simulink model "System_Design_Quadrocopter"  (Simulink 7.5)
settings: Solver=ode45  StartTime=0.0  StopTime=30  RelTol=1e-3
model workspace (MAT data in the model file):
  System_Design_Quadrocopter_optim : srogui.SimProjectForm (value not decoded)
values from neighbouring files (symbols this model uses):
  phi0 = 0.15    [Quadrocopter_control_Driver.m]    (also in calc_stability.m = 0)
  r_phi0 = 0    [Quadrocopter_control_Driver.m]    (also in calc_stability.m)
  r_psi0 = 0    [Quadrocopter_control_Driver.m]    (also in calc_stability.m)
  r_theta0 = 0    [Quadrocopter_control_Driver.m]    (also in calc_stability.m)
  theta0 = 0.15    [Quadrocopter_control_Driver.m]    (also in calc_stability.m = 0)
  Ts = 0.01    [Reglerauslegung.m]    (also in Test_Reglerauslegung.m)
undefined symbols (not defined in the file or in its folder): bodyCtrl_phiCtrl_KD, bodyCtrl_phiCtrl_KI, bodyCtrl_phiCtrl_KP, bodyCtrl_rphiCtrl_KD, bodyCtrl_rphiCtrl_KI, bodyCtrl_rphiCtrl_KP, bodyCtrl_rpsiCtrl_KD, bodyCtrl_rpsiCtrl_KI, bodyCtrl_rpsiCtrl_KP, bodyCtrl_rthetaCtrl_KD, bodyCtrl_rthetaCtrl_KI, bodyCtrl_rthetaCtrl_KP, bodyCtrl_thetaCtrl_KD, bodyCtrl_thetaCtrl_KI, bodyCtrl_thetaCtrl_KP, boom, f1, f2, f3, f4, f5, g, I_x, I_y, I_z, m, positionCtrl_rpsiCtrl_KD, positionCtrl_rpsiCtrl_KI, positionCtrl_rpsiCtrl_KP, sigbuilder_block, speed, thrust, Ts_Opt
libraries: simulink x39, dspobslib x4, Copter_Library x3, Control_lib x1, sdolib x1
(part 1 of 4)
CloseFcn:
  | rtwprivate ssgensfun ModelCloseRequest System_Design_Quadrocopter
settings Model: Creator=roczit00  LastModifiedBy=Anonymos  BufferReuse=off
settings DataIOCC: LimitDataPoints=off
settings OptimizationCC: BlockReduction=off  InlineParams=on  BufferReuse=off
settings DebuggingCC: AlgebraicLoopMsg=none  SolverPrmCheckMsg=none  UnconnectedInputMsg=none  UnconnectedOutputMsg=none  UnconnectedLineMsg=none  StrictBusMsg=Warning

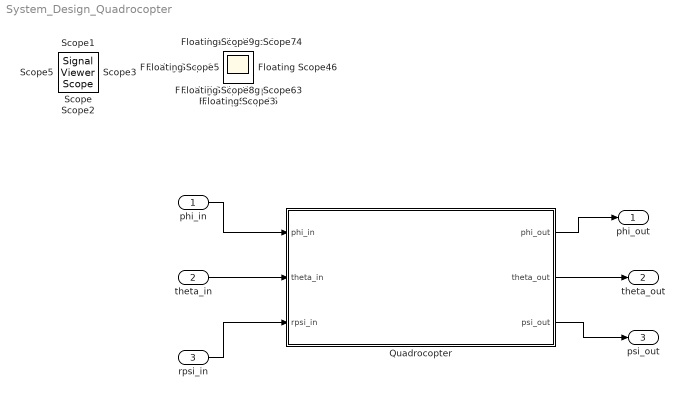
== system System_Design_Quadrocopter ==
  phi_in : Inport  OutDataType=fixdt(1, 16)  OutScaling=2^0
  theta_in : Inport  Port=2  OutDataType=fixdt(1, 16)  OutScaling=2^0
  rpsi_in : Inport  Port=3  OutDataType=fixdt(1, 16)  OutScaling=2^0
  Quadrocopter : Subsystem
  phi_out : Outport  OutDataType=fixdt(1, 16)  OutScaling=2^0
  theta_out : Outport  Port=2  OutDataType=fixdt(1, 16)  OutScaling=2^0
  psi_out : Outport  Port=3  OutDataType=fixdt(1, 16)  OutScaling=2^0
  Floating Scope{,1..18} (19 alike) : Scope
      Floating Scope settings: Floating=on  YMin=-40  YMax=90
      Floating Scope1 settings: Floating=on
      Floating Scope10 settings: Floating=on  SaveName=ScopeData12
      Floating Scope11 settings: Floating=on  SaveName=ScopeData13
      Floating Scope12 settings: Floating=on  YMin=-2500  YMax=27500  SaveName=ScopeData14
      Floating Scope13 settings: Floating=on  YMin=0  YMax=0.3  SaveName=ScopeData15
      Floating Scope14 settings: Floating=on  SaveName=ScopeData8
      Floating Scope15 settings: Floating=on  SaveName=ScopeData9
      Floating Scope16 settings: Floating=on  YMin=-0.35  YMax=0.15  SaveName=ScopeData16
      Floating Scope17 settings: Floating=on  YMin=0.1  YMax=0.55  SaveName=ScopeData17
      Floating Scope18 settings: Floating=on  SaveName=ScopeData18
      Floating Scope2 settings: Floating=on  YMin=-6000  YMax=2500  SaveName=ScopeData2
      Floating Scope3 settings: Floating=on  SaveName=ScopeData3
      Floating Scope4 settings: Floating=on  SaveName=ScopeData4
      Floating Scope5 settings: Floating=on  YMin=-0.7  YMax=0.8  SaveName=ScopeData5
      Floating Scope6 settings: Floating=on  YMin=-1  YMax=1  SaveName=ScopeData6
      Floating Scope7 settings: Floating=on  YMin=-15  YMax=10  SaveName=ScopeData7
      Floating Scope8 settings: Floating=on  YMax=45  SaveName=ScopeData10
      Floating Scope9 settings: Floating=on  YMin=-7  YMax=9  SaveName=ScopeData11
  Scope{,1..3,5} (5 alike) : SignalViewerScope  IOType=viewer  RefreshTime=0.035000
      Scope settings: YMin=-0.01  YMax=0.1
      Scope2 settings: SaveName=ScopeData2
      Scope3 settings: SaveName=ScopeData3
      Scope5 settings: YMin=0  YMax=275  SaveName=ScopeData4
  wires:
  rpsi_in/1 -> Quadrocopter/3(rpsi_in)
  theta_in/1 -> Quadrocopter/2(theta_in)
  phi_in/1 -> Quadrocopter/1(phi_in)
  Quadrocopter/1(phi_out) -> phi_out/1
  Quadrocopter/3(psi_out) -> psi_out/1
  Quadrocopter/2(theta_out) -> theta_out/1

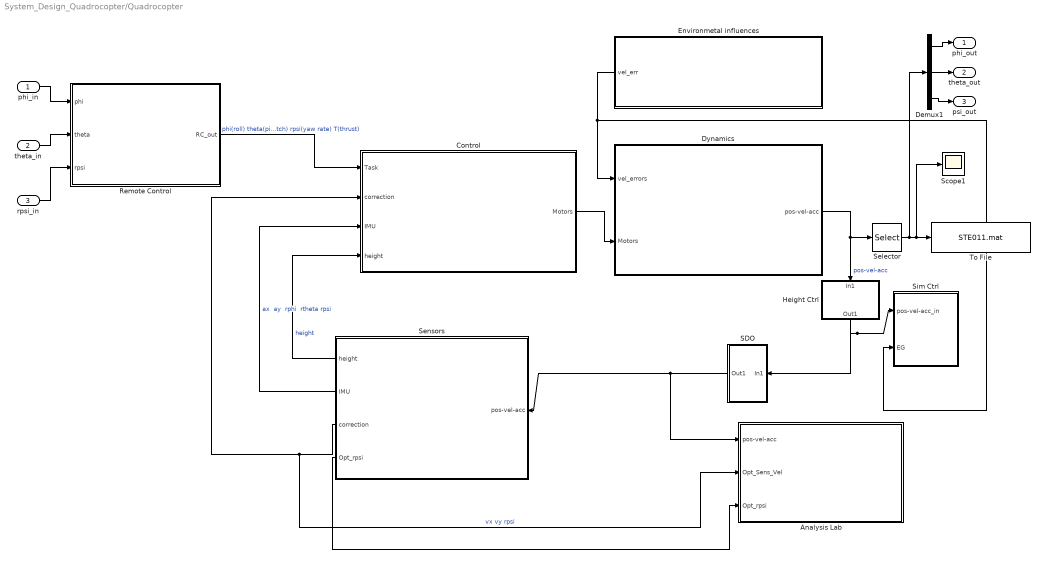
== system System_Design_Quadrocopter/Quadrocopter ==
  phi_in : Inport  OutDataType=fixdt(1, 16)  OutScaling=2^0
  theta_in : Inport  Port=2  OutDataType=fixdt(1, 16)  OutScaling=2^0
  rpsi_in : Inport  Port=3  OutDataType=fixdt(1, 16)  OutScaling=2^0
  Analysis Lab : Subsystem
      mask Display: image(imresize(imread('DecoImg/Lab.jpg'),0.12), 'center');
  Control : Subsystem
      mask Display: image(imresize(imread('DecoImg/Control.jpg'),0.2), 'center');
  Demux1 : Demux  Outputs=3
  Dynamics : Subsystem
      mask Display: image(imresize(imread('DecoImg/Dynamics.jpg'),0.2), 'center');
  Environmetal influences : Subsystem
      mask Display: image(imresize(imread('DecoImg/Environment.jpg'),0.2), 'center');
  Height Ctrl : Subsystem  mask{Step_T=0, Gain=5, Delay=3}
      mask prompts: Step_T "Step Time"; Delay "LP Delay"
  Remote Control : Subsystem
      mask Display: image(imresize(imread('DecoImg/RemoteControl.jpg'),0.3), 'center');
  SDO : Subsystem
  Scope1 : Scope
      settings: YMin=-2  YMax=2  SaveName=ScopeData22
  Selector : Selector  InputPortWidth=pos_vel_acc_dim  IndexOptions=Index vector (dialog)  Indices=[4 5 12]  OutputSizes=1
  Sensors : Subsystem
      mask Display: image(imresize(imread('DecoImg/Sensors.jpg'),0.1), 'center');
  Sim Ctrl : Subsystem  mask{Per_Cent_Gain=0.1, ErrorGain=6}
      mask prompts: Per_Cent_Gain "Per Cent of Gain for threshold"; ErrorGain "Error Gain"
  To File : ToFile  Filename=STE011.mat  MatrixName=Tfile
  phi_out : Outport  OutDataType=fixdt(1, 16)  OutScaling=2^0
  theta_out : Outport  Port=2  OutDataType=fixdt(1, 16)  OutScaling=2^0
  psi_out : Outport  Port=3  OutDataType=fixdt(1, 16)  OutScaling=2^0
  wires:
  Control/1(Motors) -> Dynamics/2(Motors)
  Dynamics/1(pos-vel-acc) -> Height Ctrl/1(In1), Selector/1  "pos-vel-acc"
  Sensors/2(IMU) -> Control/3(IMU)  "ax  ay  rphi  rtheta rpsi"
  Sensors/1(height) -> Control/4(height)  "height"
  Sensors/3(correction) -> Control/2(correction), Analysis Lab/2(Opt_Sens_Vel)  "vx vy rpsi"
  Environmetal influences/1(vel_err) -> Dynamics/1(vel_errors), Sim Ctrl/2(EG)
  Height Ctrl/1(Out1) -> Sim Ctrl/1(pos-vel-acc_in), SDO/1(In1)
  Sensors/4(Opt_rpsi) -> Analysis Lab/3(Opt_rpsi)
  Remote Control/1(RC_out) -> Control/1(Task)  "phi(roll) theta(pitch) rpsi(yaw rate) T(thrust)"
  Selector/1 -> Scope1/1, To File/1, Demux1/1
  SDO/1(Out1) -> Analysis Lab/1(pos-vel-acc), Sensors/1(pos-vel-acc)
  rpsi_in/1 -> Remote Control/3(rpsi)
  theta_in/1 -> Remote Control/2(theta)
  phi_in/1 -> Remote Control/1(phi)
  Demux1/3 -> psi_out/1
  Demux1/2 -> theta_out/1
  Demux1/1 -> phi_out/1

== system System_Design_Quadrocopter/Quadrocopter/Analysis Lab ==
  note: [Time Opt_Vx Opt_Vy Opt_Rpsi Opt_x Opt_y Opt_psi x y z vx vy rpsi]
  pos-vel-acc : Inport
  Opt_Sens_Vel : Inport  Port=2
  Opt_rpsi : Inport  Port=3
  Copter Animation : Subsystem  mask(Quadrocopter Animation){AXES=[-100 100 -100 100 0 100], T_INT=1/25, K_VAR=Feste Position, K_POS=[30 0 6], K_ANGLE=27, A_ON=on, u_phi=on, u_theta=on, u_psi=on, u_x=on, u_y=on, u_z=on}
      mask prompts: AXES "Achsen Grenzen [xmin xmax ymin ymax zmin zmax]"; T_INT "Zeitintervall zwischen Aktualisierungen [s]:"; K_VAR "Kamera Art:"; K_POS "Ort der Kamera [xc yc zc]:"; K_ANGLE "Öffnungswinkel der Kamera [Grad]:"; A_ON "Animation Einschalten:"; u_phi "Use Input phi:"; u_theta "Use Input theta:"; u_psi "Use Input psi:"; u_x "Use Input x:"; u_y "Use Input y:"; u_z "Use Input z:"
      mask help: Erstellt eine 3-D animierte Ansicht eines Quadrocopters.
      mask init:
      | Config.axes = AXES;
      | Config.update = T_INT;
      | Config.camera_view = K_VAR;
      | Config.camera_pos = K_POS;
      | Config.view = K_ANGLE;
      | Config.Animenable = A_ON;
      | Config.phi = u_phi;
      | Config.theta = u_theta;
      | Config.psi = u_psi;
      | Config.x = u_x;
      | Config.y = u_y;
      | Config.z = u_z;
      mask Help:
      | <p>Dieser Block erstellt ein 3 dimensionales Fenster eines Quadrocopters.
      | 
      | <p><H4>Block Eingänge</H4>
      | Der Eingangsvektor bestehend aus:
      | <ul>
      | <li>X-Koordinate - Ort bezogen auf die X-Achse
      | <li>Y-Koordinate - Ort bezogen auf die Y-Achse
      | <li>Z-Koordinate - Ort bezogen auf die Z-Achse
      | <li>Psi - Yaw Drehung um die Z-Achse
      | <li>Phi - Roll Drehen um die Achse in Flugrichtung
      | <li>theta - pitch Neigung in Flugrichtung nach oben bzw. unten
      | </ul></p>
      mask StyleString: edit,edit,popup(Feste Position|Frei bewegbar),edit,edit,checkbox,checkbox,checkbox,checkbox,checkbox,checkbox,checkbox
  Demux : Demux  Outputs=6
  Demux2 : Demux  Outputs=3
  Integrator1 : Integrator
  Integrator2 : Integrator
  Integrator3 : Integrator
  Mux : Mux  Inputs=3
  Mux1 : Mux  Inputs=6
  Mux3 : Mux  Inputs=3
  Selector : Selector  InputPortWidth=pos_vel_acc_dim  IndexOptions=Index vector (dialog)  Indices=[1 2 3 20 21 12]  OutputSizes=1
  To File : ToFile  Filename=Rec2013.mat  MatrixName=Tfile
  wires:
  pos-vel-acc/1 -> Selector/1, Copter Animation/1(pos_vel_acc)
  Mux/1 -> To File/1
  Selector/1 -> Demux/1
  Demux/1 -> Mux1/1
  Demux/2 -> Mux1/2
  Demux/3 -> Mux1/3
  Demux/4 -> Integrator2/1
  Demux/5 -> Integrator1/1
  Demux/6 -> Mux1/6
  Integrator1/1 -> Mux1/5
  Integrator2/1 -> Mux1/4
  Mux1/1 -> Mux/3
  Demux2/1 -> Mux3/1
  Demux2/2 -> Mux3/2
  Opt_Sens_Vel/1 -> Demux2/1
  Opt_rpsi/1 -> Mux3/3
  Mux3/1 -> Mux/1, Integrator3/1
  Integrator3/1 -> Mux/2

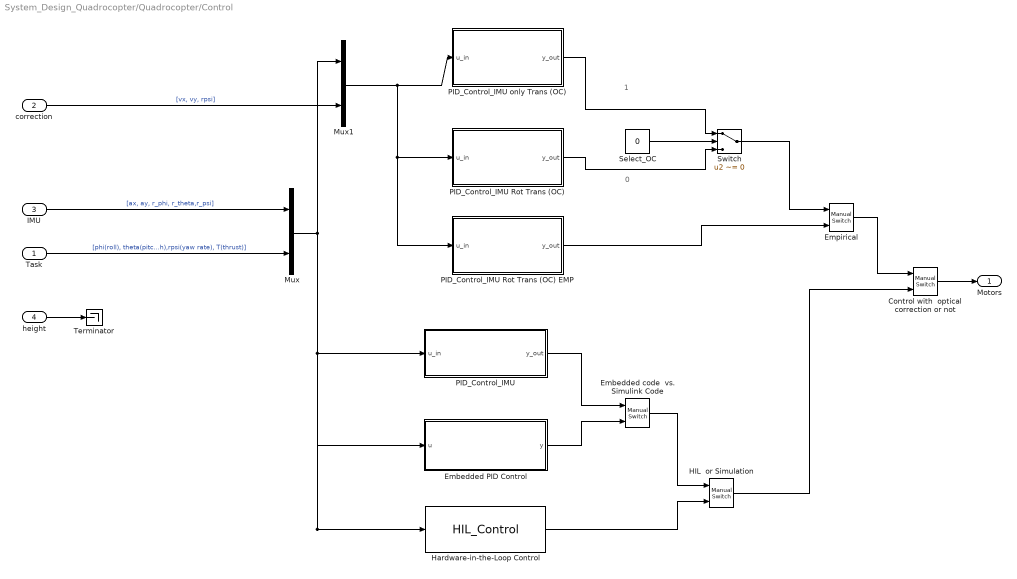
== system System_Design_Quadrocopter/Quadrocopter/Control ==
  note: 1
  note: 0
  Task : Inport  PortDimensions=4  DataType=double  OutDataTypeStr=double
  correction : Inport  Port=2
  IMU : Inport  Port=3
  height : Inport  Port=4  DataType=int16  OutDataTypeStr=int16
  Control with  optical correction or not : simulink/Signal Routing/Manual Switch  SystemSampleTime=-1  sw=1  action=0  varsize=off
  Embedded PID Control : Stateflow chart  TreatAsAtomicUnit=on
  Embedded code  vs. Simulink Code : simulink/Signal Routing/Manual Switch  SystemSampleTime=-1  sw=1  action=0  varsize=off
  Empirical : simulink/Signal Routing/Manual Switch  SystemSampleTime=-1  sw=0  action=0  varsize=off
  HIL  or Simulation : simulink/Signal Routing/Manual Switch  SystemSampleTime=-1  sw=1  action=0  varsize=off
  Hardware-in-the-Loop Control : Control_lib/HIL_Control  enabled=off
  Mux : Mux  Inputs=2
  Mux1 : Mux  Inputs=2
  PID_Control_IMU : Subsystem  AncestorBlock=Control_lib/PID_Regler
  PID_Control_IMU Rot Trans (OC) : Subsystem  AncestorBlock=Control_lib/PID_Regler  mask{set_val_th=0.1}
      mask prompts: set_val_th "Set-Value Threshold for autonomous control (set_val_th)"
  PID_Control_IMU Rot Trans (OC) EMP : Subsystem  AncestorBlock=Control_lib/PID_Regler  mask{set_val_th=0.1}
      mask prompts: set_val_th "Set-Value Threshold for autonomous control (set_val_th)"
  PID_Control_IMU only Trans (OC) : Subsystem  AncestorBlock=Control_lib/PID_Regler  mask{set_val_th=0.1}
      mask prompts: set_val_th "Set-Value Threshold for autonomous control (set_val_th)"
  Select_OC : Constant  Value=0  OutDataType=fixdt(1, 16)  OutScaling=2^0
  Switch : Switch  Criteria=u2 ~= 0  OutDataType=fixdt(1, 16)  OutScaling=2^0
  Terminator : Terminator
  Motors : Outport  PortDimensions=4
  wires:
  IMU/1 -> Mux/1  "[ax, ay, r_phi, r_theta,r_psi]"
  Task/1 -> Mux/2  "[phi(roll), theta(pitch),rpsi(yaw rate), T(thrust)]"
  height/1 -> Terminator/1
  Control with  optical correction or not/1 -> Motors/1
  Mux/1 -> Mux1/1, PID_Control_IMU/1(u_in), Embedded PID Control/1(u), Hardware-in-the-Loop Control/1
  correction/1 -> Mux1/2  "[vx, vy, rpsi]"
  HIL  or Simulation/1 -> Control with  optical correction or not/2
  Embedded code  vs. Simulink Code/1 -> HIL  or Simulation/1
  Hardware-in-the-Loop Control/1 -> HIL  or Simulation/2
  Embedded PID Control/1(y) -> Embedded code  vs. Simulink Code/2
  PID_Control_IMU/1(y_out) -> Embedded code  vs. Simulink Code/1
  Mux1/1 -> PID_Control_IMU only Trans (OC)/1(u_in), PID_Control_IMU Rot Trans (OC)/1(u_in), PID_Control_IMU Rot Trans (OC) EMP/1(u_in)
  PID_Control_IMU only Trans (OC)/1(y_out) -> Switch/1
  PID_Control_IMU Rot Trans (OC)/1(y_out) -> Switch/3
  Select_OC/1 -> Switch/2
  Switch/1 -> Empirical/1
  PID_Control_IMU Rot Trans (OC) EMP/1(y_out) -> Empirical/2
  Empirical/1 -> Control with  optical correction or not/1

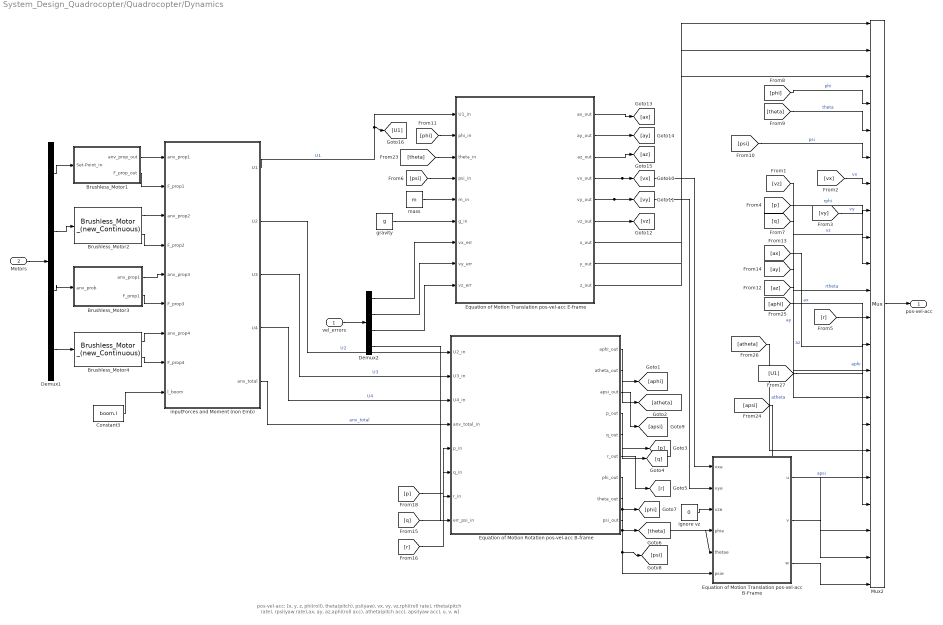
== system System_Design_Quadrocopter/Quadrocopter/Dynamics ==
  note: pos-vel-acc: [x, y, z, phi(roll), theta(pitch), psi(yaw), vx, vy, vz,rphi(roll rate), rtheta(pitch rate), rpsi(yaw rate),ax, ay, az,aphi(roll acc), atheta(pitch acc), apsi(yaw acc), u, v, w]
  vel_errors : Inport
  Motors : Inport  Port=2
  Brushless_Motor1 : Subsystem  AncestorBlock=Copter_Library/Brushless_Motor _(new_Continuous)  mask{M_error=1.01}
      mask prompts: M_error "Motor-Force pitch error [1 = no error, 0.9 = 10% negativ error, 1.1 = 10% positive error]:"
  Brushless_Motor2 : Copter_Library/Brushless_Motor _(new_Continuous)  SystemSampleTime=-1  M_error=1.01
  Brushless_Motor3 : Subsystem  AncestorBlock=Copter_Library/Brushless_Motor _(new_Continuous)  mask{M_error=1.01}
      mask prompts: M_error "Motor-Force pitch error [1 = no error, 0.9 = 10% negativ error, 1.1 = 10% positive error]:"
  Brushless_Motor4 : Copter_Library/Brushless_Motor _(new_Continuous)  SystemSampleTime=-1  M_error=1.01
  Constant3 : Constant  Value=boom.l
  Demux1 : Demux
  Demux2 : Demux
  Equation of Motion Rotation pos-vel-acc B-frame : Subsystem
  Equation of Motion Translation pos-vel-acc B-Frame : Subsystem
  Equation of Motion Translation pos-vel-acc E-frame : Subsystem
  Ignore vz : Constant  Value=0
  Mux2 : Mux  Inputs=22
  gravity : Constant  Value=g
  inputForces and Moment (non Emb) : Subsystem  AncestorBlock="Copter_Library/inputForces and  Moment (non Emb)"
  mass : Constant  Value=m
  pos-vel-acc : Outport
  wires:
  [apsi] -> Mux2/18  "apsi"
  [atheta] -> Mux2/17  "atheta"
  [aphi] -> Mux2/16  "aphi"
  [az] -> Mux2/15  "az"
  [ay] -> Mux2/14  "ay"
  [ax] -> Mux2/13  "ax"
  [q] -> Mux2/11  "rtheta"
  [p] -> Mux2/10  "rphi"
  [vz] -> Mux2/9  "vz"
  [vy] -> Mux2/8  "vy"
  [vx] -> Mux2/7  "vx"
  [psi] -> Mux2/6  "psi"
  [theta] -> Mux2/5  "theta"
  [phi] -> Mux2/4  "phi"
  Equation of Motion Translation pos-vel-acc E-frame/9(z_out) -> Mux2/3
  Motors/1 -> Demux1/1
  Demux1/3 -> Brushless_Motor3/1(anv_prob)
  Demux1/4 -> Brushless_Motor4/1
  Demux1/2 -> Brushless_Motor2/1
  Demux1/1 -> Brushless_Motor1/1(Set-Point_in)
  Constant3/1 -> inputForces and Moment (non Emb)/9(l_boom)
  inputForces and Moment (non Emb)/4(U4) -> Equation of Motion Rotation pos-vel-acc B-frame/3(U4_in)  "U4"
  inputForces and Moment (non Emb)/3(U3) -> Equation of Motion Rotation pos-vel-acc B-frame/2(U3_in)  "U3"
  inputForces and Moment (non Emb)/2(U2) -> Equation of Motion Rotation pos-vel-acc B-frame/1(U2_in)  "U2"
  Brushless_Motor1/1(anv_prop_out) -> inputForces and Moment (non Emb)/1(anv_prop1)
  Brushless_Motor1/2(F_prop_out) -> inputForces and Moment (non Emb)/2(F_prop1)
  Brushless_Motor2/1 -> inputForces and Moment (non Emb)/3(anv_prop2)
  Brushless_Motor2/2 -> inputForces and Moment (non Emb)/4(F_prop2)
  Brushless_Motor3/1(anv_prop1) -> inputForces and Moment (non Emb)/5(anv_prop3)
  Brushless_Motor3/2(F_prop1) -> inputForces and Moment (non Emb)/6(F_prop3)
  Brushless_Motor4/1 -> inputForces and Moment (non Emb)/7(anv_prop4)
  Brushless_Motor4/2 -> inputForces and Moment (non Emb)/8(F_prop4)
  Equation of Motion Translation pos-vel-acc E-frame/7(x_out) -> Mux2/1
  Equation of Motion Translation pos-vel-acc E-frame/8(y_out) -> Mux2/2
  inputForces and Moment (non Emb)/1(U1) -> [U1], Equation of Motion Translation pos-vel-acc E-frame/1(U1_in)  "U1"
  [phi] -> Equation of Motion Translation pos-vel-acc E-frame/2(phi_in)
  [theta] -> Equation of Motion Translation pos-vel-acc E-frame/3(theta_in)
  [psi] -> Equation of Motion Translation pos-vel-acc E-frame/4(psi_in)
  mass/1 -> Equation of Motion Translation pos-vel-acc E-frame/5(m_in)
  gravity/1 -> Equation of Motion Translation pos-vel-acc E-frame/6(g_in)
  [U1] -> Mux2/19
  Equation of Motion Translation pos-vel-acc E-frame/6(vz_out) -> [vz]
  Equation of Motion Translation pos-vel-acc E-frame/3(az_out) -> [az]
  Equation of Motion Translation pos-vel-acc E-frame/1(ax_out) -> [ax]
  Equation of Motion Translation pos-vel-acc E-frame/2(ay_out) -> [ay]
  inputForces and Moment (non Emb)/5(anv_total) -> Equation of Motion Rotation pos-vel-acc B-frame/4(anv_total_in)  "anv_total"
  Equation of Motion Rotation pos-vel-acc B-frame/1(aphi_out) -> [aphi]
  [q] -> Equation of Motion Rotation pos-vel-acc B-frame/6(q_in)
  [r] -> Equation of Motion Rotation pos-vel-acc B-frame/7(r_in)
  [p] -> Equation of Motion Rotation pos-vel-acc B-frame/5(p_in)
  Equation of Motion Rotation pos-vel-acc B-frame/2(atheta_out) -> [atheta]
  Equation of Motion Rotation pos-vel-acc B-frame/4(p_out) -> [p]
  Equation of Motion Rotation pos-vel-acc B-frame/5(q_out) -> [q]
  Equation of Motion Rotation pos-vel-acc B-frame/7(phi_out) -> [phi], Equation of Motion Translation pos-vel-acc B-Frame/4(phie)
  Equation of Motion Rotation pos-vel-acc B-frame/8(theta_out) -> [theta], Equation of Motion Translation pos-vel-acc B-Frame/5(thetae)
  Equation of Motion Rotation pos-vel-acc B-frame/9(psi_out) -> [psi], Equation of Motion Translation pos-vel-acc B-Frame/6(psie)
  Demux2/1 -> Equation of Motion Translation pos-vel-acc E-frame/7(vx_err)
  Demux2/2 -> Equation of Motion Translation pos-vel-acc E-frame/8(vy_err)
  Demux2/3 -> Equation of Motion Translation pos-vel-acc E-frame/9(vz_err)
  vel_errors/1 -> Demux2/1
  Mux2/1 -> pos-vel-acc/1
  Equation of Motion Translation pos-vel-acc E-frame/4(vx_out) -> [vx], Equation of Motion Translation pos-vel-acc B-Frame/1(vxe)
  Equation of Motion Translation pos-vel-acc E-frame/5(vy_out) -> [vy], Equation of Motion Translation pos-vel-acc B-Frame/2(vye)
  Ignore vz/1 -> Equation of Motion Translation pos-vel-acc B-Frame/3(vze)
  Equation of Motion Translation pos-vel-acc B-Frame/1(u) -> Mux2/20
  Equation of Motion Translation pos-vel-acc B-Frame/2(v) -> Mux2/21
  Equation of Motion Translation pos-vel-acc B-Frame/3(w) -> Mux2/22
  Demux2/4 -> Equation of Motion Rotation pos-vel-acc B-frame/8(err_psi_in)
  Equation of Motion Rotation pos-vel-acc B-frame/3(apsi_out) -> [apsi]
  Equation of Motion Rotation pos-vel-acc B-frame/6(r_out) -> [r]
  [r] -> Mux2/12

== system System_Design_Quadrocopter/Quadrocopter/Environmetal influences ==
  Mux1 : Mux
  Step_r_psi_E_error : Step  Time=[5]  After=[1]  SampleTime=0
  Step_v_x_E_error : Step  Time=[5]  After=0  SampleTime=0
  Step_v_y_E_error : Step  Time=[5]  After=[0]  SampleTime=0
  Step_v_z_E_error : Step  Time=[0]  After=[0]  SampleTime=0
  vel_err : Outport
  wires:
  Mux1/1 -> vel_err/1
  Step_v_y_E_error/1 -> Mux1/2
  Step_v_z_E_error/1 -> Mux1/3
  Step_v_x_E_error/1 -> Mux1/1
  Step_r_psi_E_error/1 -> Mux1/4

== system System_Design_Quadrocopter/Quadrocopter/Height Ctrl ==
  note: pos-vel-acc: [x, y, z, phi(roll), theta(pitch), psi(yaw), vx, vy, vz,rphi(roll rate), rtheta(pitch rate), rpsi(yaw rate),ax, ay, az,aphi(roll acc), atheta(pitch acc), apsi(yaw acc), u, v, w]
  In1 : Inport  OutDataType=fixdt(1, 16)  OutScaling=2^0
  Delay : TransferFcn  Denominator=[Delay 1]  ContinuousStateAttributes='Motor_Delay'
  Demux : Demux  Outputs=pos_vel_acc_dim
  Integrator : Integrator
  Integrator1 : Integrator
  Mux2 : Mux  Inputs=pos_vel_acc_dim
  Step : Step  Time=Step_T  After=Gain  SampleTime=0
  Terminator : Terminator
  Terminator1 : Terminator
  Terminator2 : Terminator
  Out1 : Outport
  wires:
  Step/1 -> Delay/1
  Demux/1 -> Mux2/1
  Demux/2 -> Mux2/2
  Demux/4 -> Mux2/4
  Demux/5 -> Mux2/5
  Demux/6 -> Mux2/6
  Demux/7 -> Mux2/7
  Demux/10 -> Mux2/10
  Demux/11 -> Mux2/11
  Demux/13 -> Mux2/13
  Demux/16 -> Mux2/16
  Demux/17 -> Mux2/17
  Demux/18 -> Mux2/18
  Demux/19 -> Mux2/19
  Demux/20 -> Mux2/20
  Demux/21 -> Mux2/21
  Demux/22 -> Mux2/22
  Mux2/1 -> Out1/1
  In1/1 -> Demux/1
  Delay/1 -> Integrator/1, Mux2/3
  Integrator/1 -> Integrator1/1, Mux2/9
  Demux/8 -> Mux2/8
  Demux/3 -> Terminator2/1
  Demux/9 -> Terminator1/1
  Integrator1/1 -> Mux2/15
  Demux/15 -> Terminator/1
  Demux/14 -> Mux2/14
  Demux/12 -> Mux2/12

== system System_Design_Quadrocopter/Quadrocopter/Remote Control ==
  note: phi(roll)
      | theta(pitch)
      | rpsi(yaw rate)
      | T(thrust)
  phi : Inport  OutDataType=fixdt(1, 16)  OutScaling=2^0
  theta : Inport  Port=2  OutDataType=fixdt(1, 16)  OutScaling=2^0
  rpsi : Inport  Port=3  OutDataType=fixdt(1, 16)  OutScaling=2^0
  3D-Mouse : simulink/Signal Routing/Manual Switch  SystemSampleTime=-1  sw=0  action=0  varsize=off
  Allow 3D Mouse : dspobslib/DSP Constant  SystemSampleTime=-1  Value=1  SampleMode=Discrete  discreteOutput=Sample-based  continuousOutput=Sample-based  sampTime=inf  framePeriod=2  dataType=boolean  isSigned=on  wordLen=16  udDataType=sfix(16)  fracBitsMode=Best precision  numFracBits=15  InterpretAs1D=-inf  Ts=-inf  FramebasedOutput=-inf
  Const or Square : simulink/Signal Routing/Manual Switch  SystemSampleTime=-1  sw=1  action=0  varsize=off
  Const_Stimuli : Subsystem  AncestorBlock=Remote_Control_Library/Remote_Control_Pitch_stimuli
  Disable 3D Mouse : dspobslib/DSP Constant  SystemSampleTime=-1  Value=0  SampleMode=Discrete  discreteOutput=Sample-based  continuousOutput=Sample-based  sampTime=inf  framePeriod=2  dataType=boolean  isSigned=on  wordLen=16  udDataType=sfix(16)  fracBitsMode=Best precision  numFracBits=15  InterpretAs1D=-inf  Ts=-inf  FramebasedOutput=-inf
  Mouse or Stimuli : simulink/Signal Routing/Manual Switch  SystemSampleTime=-1  sw=1  action=0  varsize=off
  Remote_Control_3d_mouse : Subsystem  AncestorBlock=Remote_Control_Library/Remote_Control_3d_mouse
  Square_path_stimuli : Subsystem  AncestorBlock=Remote_Control_Library/Remote_Control_Pitch_stimuli
  Step or Const or Square : simulink/Signal Routing/Manual Switch  SystemSampleTime=-1  sw=0  action=0  varsize=off
  Step_Stimuli : Subsystem  AncestorBlock=Remote_Control_Library/Remote_Control_Pitch_stimuli
  RC_out : Outport
  wires:
  Mouse or Stimuli/1 -> RC_out/1
  Allow 3D Mouse/1 -> 3D-Mouse/1
  Disable 3D Mouse/1 -> 3D-Mouse/2
  3D-Mouse/1 -> Remote_Control_3d_mouse/Enable
  Remote_Control_3d_mouse/1(Out1) -> Mouse or Stimuli/2
  Const_Stimuli/1(Out) -> Const or Square/1
  Square_path_stimuli/1(Out) -> Const or Square/2
  Step_Stimuli/1(Out) -> Step or Const or Square/1
  Const or Square/1 -> Step or Const or Square/2
  Step or Const or Square/1 -> Mouse or Stimuli/1
  phi/1 -> Const_Stimuli/1(phi)
  theta/1 -> Const_Stimuli/2(theta)
  rpsi/1 -> Const_Stimuli/3(rpsi)

== system System_Design_Quadrocopter/Quadrocopter/SDO ==
  note: pos-vel-acc: [x, y, z, phi(roll), theta(pitch), psi(yaw), vx, vy, vz,rphi(roll rate), rtheta(pitch rate), rpsi(yaw rate),ax, ay, az,aphi(roll acc), atheta(pitch acc), apsi(yaw acc), u, v, w]
  In1 : Inport  OutDataType=fixdt(1, 16)  OutScaling=2^0
  Demux : Demux  Outputs=pos_vel_acc_dim
  Mux2 : Mux  Inputs=pos_vel_acc_dim
  Signal Constraint : sdolib/Signal Constraint  SystemSampleTime=-1  DialogPosition=[0.0472222222222222 0.448888888888889 0.447222222222222 0.31]  SaveIn=model workspace  SaveAs=System_Design_Quadrocopter_optim  LogID=SRO_DataLog_1  Ylim=[-2 2]  SavePathFormat=absolute
  captrPsi : Subsystem
      mask init:
      | set_param('System_Design_Quadrocopter/Quadrocopter/SDO/captrPsi/cntr', 'value',num2str(get_param('System_Design_Quadrocopter/Quadrocopter/SDO/captrPsi/cntr', 'value')+1))
      | set_param('System_Design_Quadrocopter/Quadrocopter/SDO/captrPsi/To File','File name',strcat('SDO_',get_param('System_Design_Quadrocopter/Quadrocopter/SDO/captrPsi/cntr', 'value'),'.mat'))
  Out1 : Outport
  wires:
  Demux/1 -> Mux2/1
  Demux/2 -> Mux2/2
  Demux/4 -> Mux2/4
  Demux/5 -> Mux2/5
  Demux/6 -> Mux2/6
  Demux/7 -> Mux2/7
  Demux/10 -> Mux2/10
  Demux/11 -> Mux2/11
  Demux/13 -> Mux2/13
  Demux/16 -> Mux2/16
  Demux/17 -> Mux2/17
  Demux/18 -> Mux2/18
  Demux/19 -> Mux2/19
  Demux/20 -> Mux2/20
  Demux/21 -> Mux2/21
  Demux/22 -> Mux2/22
  Mux2/1 -> Out1/1
  In1/1 -> Demux/1
  Demux/8 -> Mux2/8
  Demux/14 -> Mux2/14
  Demux/12 -> Signal Constraint/1, Mux2/12, captrPsi/1(In2)
  Demux/9 -> Mux2/9
  Demux/15 -> Mux2/15
  Demux/3 -> Mux2/3

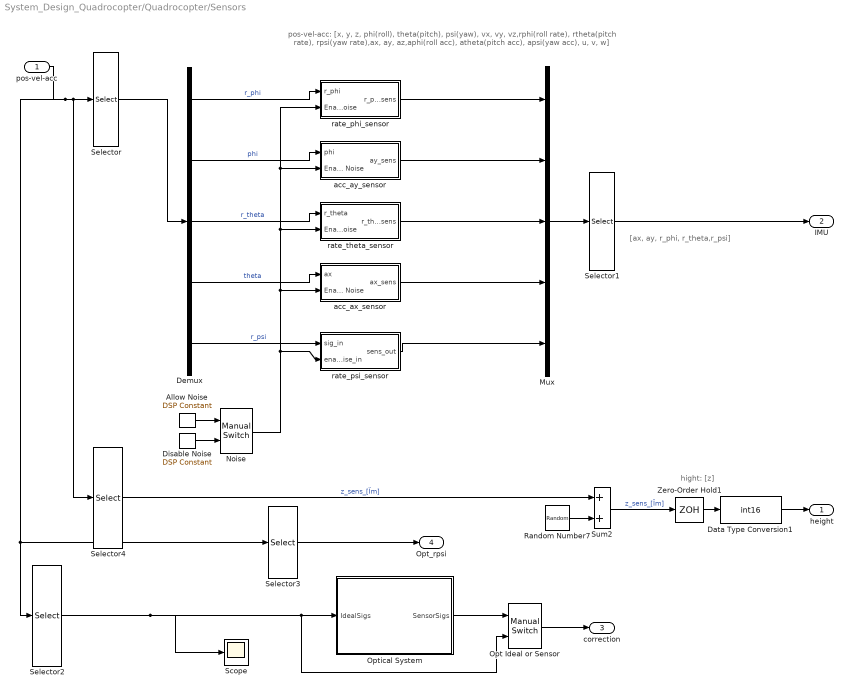
== system System_Design_Quadrocopter/Quadrocopter/Sensors ==
  note: hight: [z]
  note: pos-vel-acc: [x, y, z, phi(roll), theta(pitch), psi(yaw), vx, vy, vz,rphi(roll rate), rtheta(pitch rate), rpsi(yaw rate),ax, ay, az,aphi(roll acc), atheta(pitch acc), apsi(yaw acc), u, v, w]
  note: [ax, ay, r_phi, r_theta,r_psi]
  pos-vel-acc : Inport
  Allow Noise : dspobslib/DSP Constant  SystemSampleTime=-1  Value=1  SampleMode=Discrete  discreteOutput=Sample-based  continuousOutput=Sample-based  sampTime=inf  framePeriod=2  dataType=boolean  isSigned=on  wordLen=16  udDataType=sfix(16)  fracBitsMode=Best precision  numFracBits=15  InterpretAs1D=-inf  Ts=-inf  FramebasedOutput=-inf
  Data Type Conversion1 : DataTypeConversion  OutDataTypeMode=int16  OutDataTypeStr=int16  RndMeth=Round
  Demux : Demux  Outputs=5
  Disable Noise : dspobslib/DSP Constant  SystemSampleTime=-1  Value=0  SampleMode=Discrete  discreteOutput=Sample-based  continuousOutput=Sample-based  sampTime=inf  framePeriod=2  dataType=boolean  isSigned=on  wordLen=16  udDataType=sfix(16)  fracBitsMode=Best precision  numFracBits=15  InterpretAs1D=-inf  Ts=-inf  FramebasedOutput=-inf
  Mux : Mux  Inputs=5
  Noise : simulink/Signal Routing/Manual Switch  SystemSampleTime=-1  sw=1  action=0  varsize=off
  Opt Ideal or Sensor : simulink/Signal Routing/Manual Switch  SystemSampleTime=-1  sw=1  action=0  varsize=off
  Optical System : Subsystem  mask{Opt_Var_Trans=0.00013, Opt_Var_Rot=0.00023, Opt_Var_ST_Trans=0.001, Opt_Var_ST_Rot=0.001, Opt_Limit_Trans=5, Opt_Limit_Rot=2*pi, Opt_Delay_Global=0.1, Opt_ST_Global=0.1, Opt_Ori_SG_Trans=0.5, Opt_Ori_SG_Rot=0.2, Opt_Sens_Rec=[0.14,0.001,4,1,0.4,0.1,3.2,5,0.01,0.04]}
      mask prompts: Opt_Var_Trans "Variance of Translation"; Opt_Var_Rot "Variance of Rotation"; Opt_Var_ST_Trans "Sample Time of Variance (Translation)"; Opt_Var_ST_Rot "Sample Time of Variance (Roatation)"; Opt_Limit_Trans "Limitation [m/s] (Translation)"; Opt_Limit_Rot "Limitation [m/s] (Rotation)"; Opt_Delay_Global "Delay"; Opt_ST_Global "Sample Time (1/Frame Rate)"; Opt_Ori_SG_Trans "Original Signal Gain (Translation)"; Opt_Ori_SG_Rot "Original Signal Gain (Rotation)"; Opt_Sens_Rec "Optical All Vector"
      mask TabNameString: Translation,Rotation,Translation,Rotation,Translation,Rotation,General,General,Translation,Rotation,Rotation
  Random Number7 : RandomNumber  Variance=3.0462e-8  Seed=5756  SampleTime=0.01
  Scope : Scope
      settings: YMin=-17.5  YMax=17.5  SaveName=ScopeData27
  Selector : Selector  InputPortWidth=pos_vel_acc_dim  IndexOptions=Index vector (dialog)  Indices=[10 4 11 5 12]  OutputSizes=1
  Selector1 : Selector  InputPortWidth=5  IndexOptions=Index vector (dialog)  Indices=[4 2 1 3 5]  OutputSizes=1
  Selector2 : Selector  InputPortWidth=pos_vel_acc_dim  IndexOptions=Index vector (dialog)  Indices=[20 21 6 ]  OutputSizes=1
  Selector3 : Selector  InputPortWidth=pos_vel_acc_dim  IndexOptions=Index vector (dialog)  Indices=[12]  OutputSizes=1
  Selector4 : Selector  InputPortWidth=pos_vel_acc_dim  IndexOptions=Index vector (dialog)  Indices=[3]  OutputSizes=1
  Sum2 : Sum
  Zero-Order Hold1 : ZeroOrderHold  SampleTime=Ts
  acc_ax_sensor : Subsystem
  acc_ay_sensor : Subsystem
  rate_phi_sensor : Subsystem
  rate_psi_sensor : Subsystem
  rate_theta_sensor : Subsystem
  height : Outport
  IMU : Outport  Port=2
  correction : Outport  Port=3
  Opt_rpsi : Outport  Port=4
  wires:
  pos-vel-acc/1 -> Selector/1, Selector4/1, Selector2/1, Selector3/1
  Selector/1 -> Demux/1
  rate_phi_sensor/1(r_phi_sens) -> Mux/1
  acc_ay_sensor/1(ay_sens) -> Mux/2
  rate_theta_sensor/1(r_theta_sens) -> Mux/3
  acc_ax_sensor/1(ax_sens) -> Mux/4
  rate_psi_sensor/1(sens_out) -> Mux/5
  Demux/1 -> rate_phi_sensor/1(r_phi)  "r_phi"
  Demux/2 -> acc_ay_sensor/1(phi)  "phi"
  Demux/3 -> rate_theta_sensor/1(r_theta)  "r_theta"
  Demux/4 -> acc_ax_sensor/1(ax)  "theta"
  Demux/5 -> rate_psi_sensor/1(sig_in)  "r_psi"
  Mux/1 -> Selector1/1
  Selector1/1 -> IMU/1
  Allow Noise/1 -> Noise/1
  Disable Noise/1 -> Noise/2
  Noise/1 -> rate_psi_sensor/2(enable_noise_in), acc_ax_sensor/2(Enable Noise), rate_theta_sensor/2(Enable Noise), acc_ay_sensor/2(Enable Noise), rate_phi_sensor/2(Enable Noise)
  Selector4/1 -> Sum2/1  "z_sens_[Ïm]"
  Zero-Order Hold1/1 -> Data Type Conversion1/1
  Data Type Conversion1/1 -> height/1
  Selector2/1 -> Scope/1, Optical System/1(IdealSigs), Opt Ideal or Sensor/2
  Sum2/1 -> Zero-Order Hold1/1  "z_sens_[Ïm]"
  Random Number7/1 -> Sum2/2
  Selector3/1 -> Opt_rpsi/1
  Optical System/1(SensorSigs) -> Opt Ideal or Sensor/1
  Opt Ideal or Sensor/1 -> correction/1

== system System_Design_Quadrocopter/Quadrocopter/Sim Ctrl ==
  note: pos-vel-acc: [x, y, z, phi(roll), theta(pitch), psi(yaw), vx, vy, vz,rphi(roll rate), rtheta(pitch rate), rpsi(yaw rate),ax, ay, az,aphi(roll acc), atheta(pitch acc), apsi(yaw acc), u, v, w]
  pos-vel-acc_in : Inport  OutDataType=fixdt(1, 16)  OutScaling=2^0
  EG : Inport  Port=2  OutDataType=fixdt(1, 16)  OutScaling=2^0
  Abs : Abs  OutDataType=fixdt(1, 16)  OutScaling=2^0
  Constant : Constant  Value=Per_Cent_Gain  OutDataType=fixdt(1, 16)  OutScaling=2^0
  Embedded MATLAB Function : Stateflow chart  TreatAsAtomicUnit=on
  Embedded MATLAB Function1 : Stateflow chart  TreatAsAtomicUnit=on
  Mux : Mux  Inputs=2
  Scope : Scope
      settings: YMin=-3  YMax=6  SaveName=ScopeData24
  Selector : Selector  InputPortWidth=pos_vel_acc_dim  IndexOptions=Index vector (dialog)  Indices=[7 8 12]  OutputSizes=1
  Stop Simulation : Stop
  wires:
  pos-vel-acc_in/1 -> Selector/1
  EG/1 -> Embedded MATLAB Function/1(ErrorGains), Embedded MATLAB Function1/1(ErrorGains)
  Constant/1 -> Embedded MATLAB Function/2(perCent)
  Selector/1 -> Mux/2, Scope/1
  Embedded MATLAB Function/1(threshold) -> Mux/1
  Mux/1 -> Abs/1
  Embedded MATLAB Function1/1(ret) -> Stop Simulation/1
  Abs/1 -> Embedded MATLAB Function1/2(u)

== system System_Design_Quadrocopter/Quadrocopter/Analysis Lab/Copter Animation ==
  pos_vel_acc : Inport
  S-Function : S-Function  FunctionName=Copter_Animation  Parameters=Config  EnableBusSupport=off
  Selector2 : Selector  InputPortWidth=pos_vel_acc_dim  IndexOptions=Index vector (dialog)  Indices=[1 2 3 4 5 6]  OutputSizes=1
  wires:
  pos_vel_acc/1 -> Selector2/1
  Selector2/1 -> S-Function/1

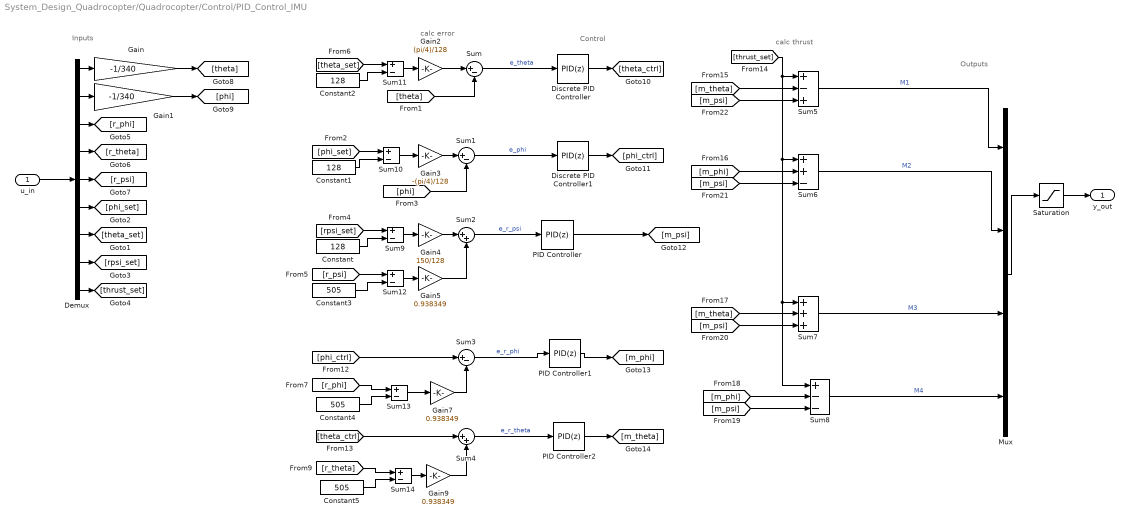
== system System_Design_Quadrocopter/Quadrocopter/Control/PID_Control_IMU ==
  note: calc thrust
  note: Control
  note: Outputs
  note: calc error
  note: Inputs
  u_in : Inport  OutDataType=fixdt(1, 16)  OutScaling=2^0
  Constant : Constant  Value=128  OutDataType=fixdt(1, 16)  OutScaling=2^0
  Constant1 : Constant  Value=128  OutDataType=fixdt(1, 16)  OutScaling=2^0
  Constant2 : Constant  Value=128  OutDataType=fixdt(1, 16)  OutScaling=2^0
  Constant3 : Constant  Value=505  OutDataType=fixdt(1, 16)  OutScaling=2^0
  Constant4 : Constant  Value=505  OutDataType=fixdt(1, 16)  OutScaling=2^0
  Constant5 : Constant  Value=505  OutDataType=fixdt(1, 16)  OutScaling=2^0
  Demux : Demux  Outputs=9
  Discrete PID Controller : simulink/Continuous/PID Controller  DialogController=pidpack.PIDConfig.pidDDGCreate  DialogControllerArgs=DataTag1  SystemSampleTime=-1  Controller=PID  TimeDomain=Discrete-time  SampleTime=Ts  IntegratorMethod=Forward Euler  FilterMethod=Forward Euler  Form=Ideal  P=150  I=0.5  D=0  N=1  InitialConditionSource=internal  InitialConditionForIntegrator=0  InitialConditionForFilter=0  ExternalReset=none  ZeroCross=off  LimitOutput=off  UpperSaturationLimit=inf  LowerSaturationLimit=-inf  LinearizeAsGain=off  AntiWindupMode=none  Kb=1  TrackingMode=off  Kt=1  PParamMin=[]  PParamMax=[]  IParamMin=[]  IParamMax=[]  DParamMin=[]  DParamMax=[]  NParamMin=[]  NParamMax=[]  KbParamMin=[]  KbParamMax=[]  KtParamMin=[]  KtParamMax=[]  POutMin=[]  POutMax=[]  IOutMin=[]  IOutMax=[]  DOutMin=[]  DOutMax=[]  NOutMin=[]  NOutMax=[]  KbOutMin=[]  KbOutMax=[]  KtOutMin=[]  KtOutMax=[]  IntegratorOutMin=[]  IntegratorOutMax=[]  FilterOutMin=[]  FilterOutMax=[]  SumOutMin=[]  SumOutMax=[]  SumI1OutMin=[]  SumI1OutMax=[]  SumI2OutMin=[]  SumI2OutMax=[]  SumI3OutMin=[]  SumI3OutMax=[]  SumDOutMin=[]  SumDOutMax=[]  SaturationOutMin=[]  SaturationOutMax=[]  IntegratorContinuousStateAttributes=''  IntegratorStateMustResolveToSignalObject=off  IntegratorRTWStateStorageClass=Auto  FilterContinuousStateAttributes=''  FilterStateMustResolveToSignalObject=off  FilterRTWStateStorageClass=Auto
  Discrete PID Controller1 : simulink/Continuous/PID Controller  DialogController=pidpack.PIDConfig.pidDDGCreate  DialogControllerArgs=DataTag2  SystemSampleTime=-1  Controller=PID  TimeDomain=Discrete-time  SampleTime=Ts  IntegratorMethod=Forward Euler  FilterMethod=Forward Euler  Form=Ideal  P=150  I=0.5  D=0  N=1  InitialConditionSource=internal  InitialConditionForIntegrator=0  InitialConditionForFilter=0  ExternalReset=none  ZeroCross=off  LimitOutput=off  UpperSaturationLimit=inf  LowerSaturationLimit=-inf  LinearizeAsGain=off  AntiWindupMode=none  Kb=1  TrackingMode=off  Kt=1  PParamMin=[]  PParamMax=[]  IParamMin=[]  IParamMax=[]  DParamMin=[]  DParamMax=[]  NParamMin=[]  NParamMax=[]  KbParamMin=[]  KbParamMax=[]  KtParamMin=[]  KtParamMax=[]  POutMin=[]  POutMax=[]  IOutMin=[]  IOutMax=[]  DOutMin=[]  DOutMax=[]  NOutMin=[]  NOutMax=[]  KbOutMin=[]  KbOutMax=[]  KtOutMin=[]  KtOutMax=[]  IntegratorOutMin=[]  IntegratorOutMax=[]  FilterOutMin=[]  FilterOutMax=[]  SumOutMin=[]  SumOutMax=[]  SumI1OutMin=[]  SumI1OutMax=[]  SumI2OutMin=[]  SumI2OutMax=[]  SumI3OutMin=[]  SumI3OutMax=[]  SumDOutMin=[]  SumDOutMax=[]  SaturationOutMin=[]  SaturationOutMax=[]  IntegratorContinuousStateAttributes=''  IntegratorStateMustResolveToSignalObject=off  IntegratorRTWStateStorageClass=Auto  FilterContinuousStateAttributes=''  FilterStateMustResolveToSignalObject=off  FilterRTWStateStorageClass=Auto
  Gain : Gain  Gain=-1/340  ParameterDataType=fixdt(1, 16)  ParameterScaling=2^0  OutDataType=fixdt(1, 16)  OutScaling=2^0
  Gain1 : Gain  Gain=-1/340  ParameterDataType=fixdt(1, 16)  ParameterScaling=2^0  OutDataType=fixdt(1, 16)  OutScaling=2^0
  Gain2 : Gain  Gain=(pi/4)/128  ParameterDataType=fixdt(1, 16)  ParameterScaling=2^0  OutDataType=fixdt(1, 16)  OutScaling=2^0
  Gain3 : Gain  Gain=-(pi/4)/128  ParameterDataType=fixdt(1, 16)  ParameterScaling=2^0  OutDataType=fixdt(1, 16)  OutScaling=2^0
  Gain4 : Gain  Gain=150/128  ParameterDataType=fixdt(1, 16)  ParameterScaling=2^0  OutDataType=fixdt(1, 16)  OutScaling=2^0
  Gain5 : Gain  Gain=0.938349  ParameterDataType=fixdt(1, 16)  ParameterScaling=2^0  OutDataType=fixdt(1, 16)  OutScaling=2^0
  Gain7 : Gain  Gain=0.938349  ParameterDataType=fixdt(1, 16)  ParameterScaling=2^0  OutDataType=fixdt(1, 16)  OutScaling=2^0
  Gain9 : Gain  Gain=0.938349  ParameterDataType=fixdt(1, 16)  ParameterScaling=2^0  OutDataType=fixdt(1, 16)  OutScaling=2^0
  Mux : Mux
  PID Controller : simulink/Continuous/PID Controller  DialogController=pidpack.PIDConfig.pidDDGCreate  DialogControllerArgs=DataTag3  SystemSampleTime=-1  Controller=PID  TimeDomain=Discrete-time  SampleTime=Ts  IntegratorMethod=Forward Euler  FilterMethod=Forward Euler  Form=Ideal  P=60  I=0.5  D=0  N=0  InitialConditionSource=internal  InitialConditionForIntegrator=0  InitialConditionForFilter=0  ExternalReset=none  ZeroCross=off  LimitOutput=off  UpperSaturationLimit=inf  LowerSaturationLimit=-inf  LinearizeAsGain=off  AntiWindupMode=none  Kb=1  TrackingMode=off  Kt=1  PParamMin=[]  PParamMax=[]  IParamMin=[]  IParamMax=[]  DParamMin=[]  DParamMax=[]  NParamMin=[]  NParamMax=[]  KbParamMin=[]  KbParamMax=[]  KtParamMin=[]  KtParamMax=[]  POutMin=[]  POutMax=[]  IOutMin=[]  IOutMax=[]  DOutMin=[]  DOutMax=[]  NOutMin=[]  NOutMax=[]  KbOutMin=[]  KbOutMax=[]  KtOutMin=[]  KtOutMax=[]  IntegratorOutMin=[]  IntegratorOutMax=[]  FilterOutMin=[]  FilterOutMax=[]  SumOutMin=[]  SumOutMax=[]  SumI1OutMin=[]  SumI1OutMax=[]  SumI2OutMin=[]  SumI2OutMax=[]  SumI3OutMin=[]  SumI3OutMax=[]  SumDOutMin=[]  SumDOutMax=[]  SaturationOutMin=[]  SaturationOutMax=[]  IntegratorContinuousStateAttributes=''  IntegratorStateMustResolveToSignalObject=off  IntegratorRTWStateStorageClass=Auto  FilterContinuousStateAttributes=''  FilterStateMustResolveToSignalObject=off  FilterRTWStateStorageClass=Auto
  PID Controller1 : simulink/Continuous/PID Controller  DialogController=pidpack.PIDConfig.pidDDGCreate  DialogControllerArgs=DataTag4  SystemSampleTime=-1  Controller=PID  TimeDomain=Discrete-time  SampleTime=Ts  IntegratorMethod=Forward Euler  FilterMethod=Forward Euler  Form=Ideal  P=60  I=0.5  D=0  N=0  InitialConditionSource=internal  InitialConditionForIntegrator=0  InitialConditionForFilter=0  ExternalReset=none  ZeroCross=off  LimitOutput=off  UpperSaturationLimit=inf  LowerSaturationLimit=-inf  LinearizeAsGain=off  AntiWindupMode=none  Kb=1  TrackingMode=off  Kt=1  PParamMin=[]  PParamMax=[]  IParamMin=[]  IParamMax=[]  DParamMin=[]  DParamMax=[]  NParamMin=[]  NParamMax=[]  KbParamMin=[]  KbParamMax=[]  KtParamMin=[]  KtParamMax=[]  POutMin=[]  POutMax=[]  IOutMin=[]  IOutMax=[]  DOutMin=[]  DOutMax=[]  NOutMin=[]  NOutMax=[]  KbOutMin=[]  KbOutMax=[]  KtOutMin=[]  KtOutMax=[]  IntegratorOutMin=[]  IntegratorOutMax=[]  FilterOutMin=[]  FilterOutMax=[]  SumOutMin=[]  SumOutMax=[]  SumI1OutMin=[]  SumI1OutMax=[]  SumI2OutMin=[]  SumI2OutMax=[]  SumI3OutMin=[]  SumI3OutMax=[]  SumDOutMin=[]  SumDOutMax=[]  SaturationOutMin=[]  SaturationOutMax=[]  IntegratorContinuousStateAttributes=''  IntegratorStateMustResolveToSignalObject=off  IntegratorRTWStateStorageClass=Auto  FilterContinuousStateAttributes=''  FilterStateMustResolveToSignalObject=off  FilterRTWStateStorageClass=Auto
  PID Controller2 : simulink/Continuous/PID Controller  DialogController=pidpack.PIDConfig.pidDDGCreate  DialogControllerArgs=DataTag5  SystemSampleTime=-1  Controller=PID  TimeDomain=Discrete-time  SampleTime=Ts  IntegratorMethod=Forward Euler  FilterMethod=Forward Euler  Form=Ideal  P=60  I=0.5  D=0  N=0  InitialConditionSource=internal  InitialConditionForIntegrator=0  InitialConditionForFilter=0  ExternalReset=none  ZeroCross=off  LimitOutput=off  UpperSaturationLimit=inf  LowerSaturationLimit=-inf  LinearizeAsGain=off  AntiWindupMode=none  Kb=1  TrackingMode=off  Kt=1  PParamMin=[]  PParamMax=[]  IParamMin=[]  IParamMax=[]  DParamMin=[]  DParamMax=[]  NParamMin=[]  NParamMax=[]  KbParamMin=[]  KbParamMax=[]  KtParamMin=[]  KtParamMax=[]  POutMin=[]  POutMax=[]  IOutMin=[]  IOutMax=[]  DOutMin=[]  DOutMax=[]  NOutMin=[]  NOutMax=[]  KbOutMin=[]  KbOutMax=[]  KtOutMin=[]  KtOutMax=[]  IntegratorOutMin=[]  IntegratorOutMax=[]  FilterOutMin=[]  FilterOutMax=[]  SumOutMin=[]  SumOutMax=[]  SumI1OutMin=[]  SumI1OutMax=[]  SumI2OutMin=[]  SumI2OutMax=[]  SumI3OutMin=[]  SumI3OutMax=[]  SumDOutMin=[]  SumDOutMax=[]  SaturationOutMin=[]  SaturationOutMax=[]  IntegratorContinuousStateAttributes=''  IntegratorStateMustResolveToSignalObject=off  IntegratorRTWStateStorageClass=Auto  FilterContinuousStateAttributes=''  FilterStateMustResolveToSignalObject=off  FilterRTWStateStorageClass=Auto
  Saturation : Saturate  UpperLimit=255  LowerLimit=0  OutDataType=fixdt(1, 16)  OutScaling=2^0
  Sum : Sum  Inputs=|+-  OutDataType=fixdt(1, 16)  OutScaling=2^0
  Sum1 : Sum  Inputs=|+-  OutDataType=fixdt(1, 16)  OutScaling=2^0
  Sum{9..14} (6 alike) : Sum  Inputs=+-  OutDataType=fixdt(1, 16)  OutScaling=2^0
  Sum2 : Sum  Inputs=|++  OutDataType=fixdt(1, 16)  OutScaling=2^0
  Sum3 : Sum  Inputs=|+-  OutDataType=fixdt(1, 16)  OutScaling=2^0
  Sum4 : Sum  Inputs=|++  OutDataType=fixdt(1, 16)  OutScaling=2^0
  Sum5 : Sum  Inputs=+-+  OutDataType=fixdt(1, 16)  OutScaling=2^0
  Sum6 : Sum  Inputs=++-  OutDataType=fixdt(1, 16)  OutScaling=2^0
  Sum7 : Sum  Inputs=+++  OutDataType=fixdt(1, 16)  OutScaling=2^0
  Sum8 : Sum  Inputs=+--  OutDataType=fixdt(1, 16)  OutScaling=2^0
  y_out : Outport  OutDataType=fixdt(1, 16)  OutScaling=2^0
  wires:
  Gain5/1 -> Sum2/2
  Sum12/1 -> Gain5/1
  Gain4/1 -> Sum2/1
  Sum9/1 -> Gain4/1
  [phi_ctrl] -> Sum3/1
  Sum14/1 -> Gain9/1
  Gain9/1 -> Sum4/2
  [theta_ctrl] -> Sum4/1
  Sum13/1 -> Gain7/1
  Gain7/1 -> Sum3/2
  Gain3/1 -> Sum1/1
  Gain2/1 -> Sum/1
  Sum11/1 -> Gain2/1
  Sum10/1 -> Gain3/1
  [r_theta] -> Sum14/1
  Constant5/1 -> Sum14/2
  [r_phi] -> Sum13/1
  Constant4/1 -> Sum13/2
  Constant3/1 -> Sum12/2
  [r_psi] -> Sum12/1
  Constant2/1 -> Sum11/2
  [theta_set] -> Sum11/1
  Constant1/1 -> Sum10/2
  [phi_set] -> Sum10/1
  Constant/1 -> Sum9/2
  [rpsi_set] -> Sum9/1
  Saturation/1 -> y_out/1
  Mux/1 -> Saturation/1
  [m_psi] -> Sum8/3
  [m_phi] -> Sum8/2
  [m_psi] -> Sum7/3
  [m_theta] -> Sum7/2
  [m_psi] -> Sum6/3
  [m_phi] -> Sum6/2
  [m_psi] -> Sum5/3
  [m_theta] -> Sum5/2
  [thrust_set] -> Sum8/1, Sum7/1, Sum6/1, Sum5/1
  PID Controller2/1 -> [m_theta]
  PID Controller1/1 -> [m_phi]
  PID Controller/1 -> [m_psi]
  Discrete PID Controller/1 -> [theta_ctrl]
  Discrete PID Controller1/1 -> [phi_ctrl]
  Sum6/1 -> Mux/2  "M2"
  Sum7/1 -> Mux/3  "M3"
  Sum8/1 -> Mux/4  "M4"
  Sum5/1 -> Mux/1  "M1"
  Sum4/1 -> PID Controller2/1  "e_r_theta"
  Sum3/1 -> PID Controller1/1  "e_r_phi"
  Sum2/1 -> PID Controller/1  "e_r_psi"
  Sum1/1 -> Discrete PID Controller1/1  "e_phi"
  [phi] -> Sum1/2
  Sum/1 -> Discrete PID Controller/1  "e_theta"
  [theta] -> Sum/2
  Gain1/1 -> [phi]
  Gain/1 -> [theta]
  Demux/9 -> [thrust_set]
  Demux/8 -> [rpsi_set]
  Demux/7 -> [theta_set]
  Demux/6 -> [phi_set]
  Demux/5 -> [r_psi]
  Demux/4 -> [r_theta]
  Demux/3 -> [r_phi]
  Demux/1 -> Gain/1
  Demux/2 -> Gain1/1
  u_in/1 -> Demux/1
